simulink model "untitled4"  (R2023b)
settings: Solver=VariableStepAuto  StartTime=0.0  StopTime=10.0  RelTol=1e-3
settings Model: Creator=LAPTOP  LastModifiedBy=LAPTOP

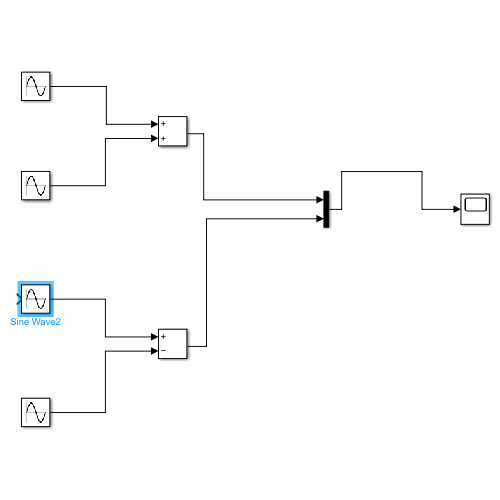
[thumbnail: Simulink's stored preview of the top-level diagram]
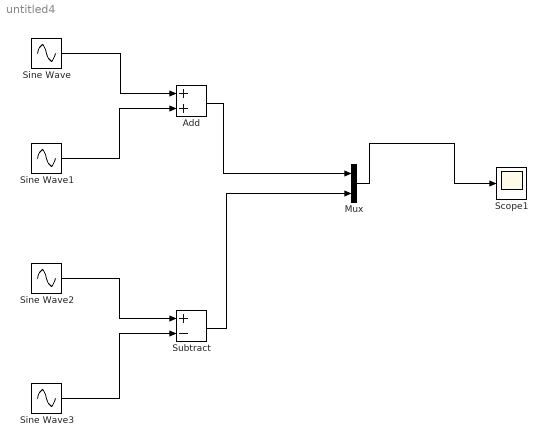
== system untitled4 ==
  Add : Sum
  Mux : Mux  Inputs=2
  Scope1 : Scope
  Sine Wave : Sin  Frequency=pi/5  SampleTime=0
  Sine Wave1 : Sin  Frequency=pi/5  Phase=pi/2  SampleTime=0
  Sine Wave2 : Sin  TimeSource=Use external signal  Frequency=pi/5  SampleTime=0
  Sine Wave3 : Sin  Frequency=pi/5  Phase=pi/2  SampleTime=0
  Subtract : Sum  Inputs=+-
  wires:
  Sine Wave/1 -> Add/1
  Sine Wave1/1 -> Add/2
  Sine Wave2/1 -> Subtract/1
  Sine Wave3/1 -> Subtract/2
  Add/1 -> Mux/1
  Subtract/1 -> Mux/2
  Mux/1 -> Scope1/1
